simulink model "ejemplosim"  (R2015a)
settings: Solver=ode45  StartTime=0.0  StopTime=7  RelTol=1e-3
settings Model: Creator=Administrador  LastModifiedBy=Administrador

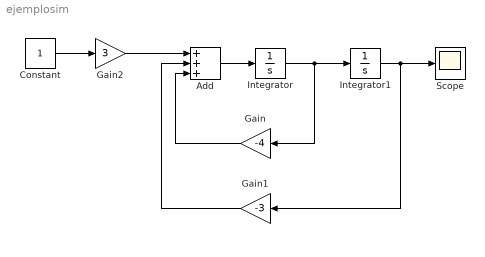
== system ejemplosim ==
  Add : Sum  Inputs=+++
  Constant : Constant
  Gain : Gain  Gain=-4
  Gain1 : Gain  Gain=-3
  Gain2 : Gain  Gain=3
  Integrator : Integrator
  Integrator1 : Integrator
  Scope : Scope
  wires:
  Integrator/1 -> Gain/1, Integrator1/1
  Add/1 -> Integrator/1
  Gain/1 -> Add/3
  Gain1/1 -> Add/2
  Constant/1 -> Gain2/1
  Gain2/1 -> Add/1
  Integrator1/1 -> Scope/1, Gain1/1
